simulink model "ami_fx_sbl_wide"  (R2012b)
settings: Solver=VariableStepDiscrete  SolverMode=SingleTasking  StartTime=0.0  StopTime=5000  RelTol=1e-3
undefined symbols (not defined in the file or in its folder): Down, Up
libraries: xbsIndex_r4 x4776, casper_library_misc x101, dspsigops x32, xps_library x23, casper_library_reorder x2, casper_library_delays x2
(part 8 of 43)

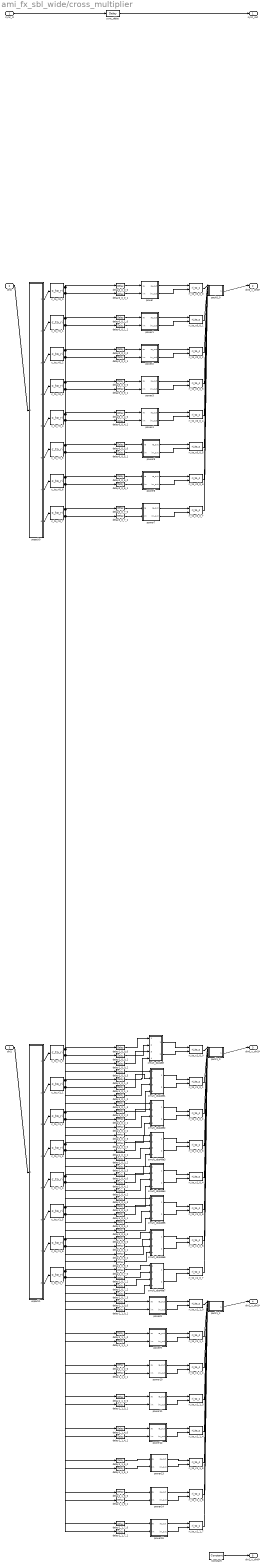
== system ami_fx_sbl_wide/cross_multiplier ==
  sync_in : Inport
  din0 : Inport  Port=2
  din1 : Inport  Port=3
  Constant : xbsIndex_r4/Constant  const=0  gui_display_data_type=Fixed-point  arith_type=Unsigned  n_bits=2*(2*bit_width_in+1)*8  bin_pt=0  preci_type=Single  exp_width=8  frac_width=24  explicit_period=on  period=1  equ=P=C  opselect=C  inp2=PCIN>>17  opr=+  inp1=P  carry=CIN  dbl_ovrd=off  block_type=constant
  c_to_ri0_{0..7} (8 alike) : casper_library_misc/c_to_ri  n_bits=bit_width_in  bin_pt=binary_point_in
  c_to_ri1_{0..7} (8 alike) : casper_library_misc/c_to_ri  n_bits=bit_width_in  bin_pt=binary_point_in
  cmult_dsp48e : Subsystem  AncestorBlock=casper_library_multipliers/cmult_dsp48e  mask(cmult_dsp48e){n_bits_a=bit_width_in, bin_pt_a=binary_point_in, n_bits_b=bit_width_in, bin_pt_b=binary_point_in, conjugated=on, full_precision=on, n_bits_c=37, bin_pt_c=34, quantization=Truncate, overflow=Wrap, cast_latency=0}
      mask prompts: n_bits_a "Bit width 'a'"; bin_pt_a "Binary point 'a'"; n_bits_b "Bit width 'b'"; bin_pt_b "Binary point 'b'"; conjugated "Conjugate"; full_precision "Full precision"; n_bits_c "Bit width out"; bin_pt_c "Binary point out"; cast_latency "Cast Latency"
      mask help:
      | Multiplies two complex numbers using 4 DSP48Es.
      | Conjugation is optional.
      |
      | Re{a} and Im{a} can be up to 25 bits.
      | Re{b} and Im{b} can be up to 18 bits.
      mask init:
      | cmult_dsp48e_init(gcb, ...
      |     'n_bits_a', n_bits_a, ...
      |     'bin_pt_a', bin_pt_a, ...
      |     'n_bits_b', n_bits_b, ...
      |     'bin_pt_b', bin_pt_b, ...
      |     'conjugated', conjugated, ...
      |     'full_precision', full_precision, ...
      |     'n_bits_c', n_bits_c, ...
      |     'bin_pt_c', bin_pt_c, ...
      |     'quantization', quantization, ...
      |     'overflow', overflow, ...
      |     'cast_latency', cast_latency);
      settings: AttributesFormatString=|
      | 18_17 * 18_17 ==> 37_34
      | Latency=4
      mask Callback full_precision:
      | full_precision = get_param(gcb, 'full_precision');
      | 
      | if strcmp(full_precision, 'on'),
      |     not_full_precision = 'off';
      | else
      |     not_full_precision = 'on';
      | end
      | 
      | set_param_state(gcb, 'n_bits_c', not_full_precision);
      | set_param_state(gcb, 'bin_pt_c', not_full_precision);
      | set_param_state(gcb, 'quantization', not_full_precision);
      | set_param_state(gcb, 'overflow', not_full_precision);
      | set_param_state(gcb, 'cast_latency', not_full_precision);
      mask TypeOptions quantization: Truncate | Round  (unbiased: +/- Inf) | Round  (unbiased: Even Values)
      mask TypeOptions overflow: Wrap | Saturate | Flag as error
  cmult_dsp48e1 : Subsystem  AncestorBlock=casper_library_multipliers/cmult_dsp48e  mask(cmult_dsp48e){n_bits_a=bit_width_in, bin_pt_a=binary_point_in, n_bits_b=bit_width_in, bin_pt_b=binary_point_in, conjugated=on, full_precision=on, n_bits_c=37, bin_pt_c=34, quantization=Truncate, overflow=Wrap, cast_latency=0}
      mask prompts: n_bits_a "Bit width 'a'"; bin_pt_a "Binary point 'a'"; n_bits_b "Bit width 'b'"; bin_pt_b "Binary point 'b'"; conjugated "Conjugate"; full_precision "Full precision"; n_bits_c "Bit width out"; bin_pt_c "Binary point out"; cast_latency "Cast Latency"
      mask help:
      | Multiplies two complex numbers using 4 DSP48Es.
      | Conjugation is optional.
      |
      | Re{a} and Im{a} can be up to 25 bits.
      | Re{b} and Im{b} can be up to 18 bits.
      mask init: same as ami_fx_sbl_wide/cross_multiplier/cmult_dsp48e
      settings: AttributesFormatString=|
      | 18_17 * 18_17 ==> 37_34
      | Latency=4
      mask Callback full_precision:
      | full_precision = get_param(gcb, 'full_precision');
      | 
      | if strcmp(full_precision, 'on'),
      |     not_full_precision = 'off';
      | else
      |     not_full_precision = 'on';
      | end
      | 
      | set_param_state(gcb, 'n_bits_c', not_full_precision);
      | set_param_state(gcb, 'bin_pt_c', not_full_precision);
      | set_param_state(gcb, 'quantization', not_full_precision);
      | set_param_state(gcb, 'overflow', not_full_precision);
      | set_param_state(gcb, 'cast_latency', not_full_precision);
      mask TypeOptions quantization: Truncate | Round  (unbiased: +/- Inf) | Round  (unbiased: Even Values)
      mask TypeOptions overflow: Wrap | Saturate | Flag as error
  cmult_dsp48e2 : Subsystem  AncestorBlock=casper_library_multipliers/cmult_dsp48e  mask(cmult_dsp48e){n_bits_a=bit_width_in, bin_pt_a=binary_point_in, n_bits_b=bit_width_in, bin_pt_b=binary_point_in, conjugated=on, full_precision=on, n_bits_c=37, bin_pt_c=34, quantization=Truncate, overflow=Wrap, cast_latency=0}
      mask prompts: n_bits_a "Bit width 'a'"; bin_pt_a "Binary point 'a'"; n_bits_b "Bit width 'b'"; bin_pt_b "Binary point 'b'"; conjugated "Conjugate"; full_precision "Full precision"; n_bits_c "Bit width out"; bin_pt_c "Binary point out"; cast_latency "Cast Latency"
      mask help:
      | Multiplies two complex numbers using 4 DSP48Es.
      | Conjugation is optional.
      |
      | Re{a} and Im{a} can be up to 25 bits.
      | Re{b} and Im{b} can be up to 18 bits.
      mask init: same as ami_fx_sbl_wide/cross_multiplier/cmult_dsp48e
      settings: AttributesFormatString=|
      | 18_17 * 18_17 ==> 37_34
      | Latency=4
      mask Callback full_precision:
      | full_precision = get_param(gcb, 'full_precision');
      | 
      | if strcmp(full_precision, 'on'),
      |     not_full_precision = 'off';
      | else
      |     not_full_precision = 'on';
      | end
      | 
      | set_param_state(gcb, 'n_bits_c', not_full_precision);
      | set_param_state(gcb, 'bin_pt_c', not_full_precision);
      | set_param_state(gcb, 'quantization', not_full_precision);
      | set_param_state(gcb, 'overflow', not_full_precision);
      | set_param_state(gcb, 'cast_latency', not_full_precision);
      mask TypeOptions quantization: Truncate | Round  (unbiased: +/- Inf) | Round  (unbiased: Even Values)
      mask TypeOptions overflow: Wrap | Saturate | Flag as error
  cmult_dsp48e3 : Subsystem  AncestorBlock=casper_library_multipliers/cmult_dsp48e  mask(cmult_dsp48e){n_bits_a=bit_width_in, bin_pt_a=binary_point_in, n_bits_b=bit_width_in, bin_pt_b=binary_point_in, conjugated=on, full_precision=on, n_bits_c=37, bin_pt_c=34, quantization=Truncate, overflow=Wrap, cast_latency=0}
      mask prompts: n_bits_a "Bit width 'a'"; bin_pt_a "Binary point 'a'"; n_bits_b "Bit width 'b'"; bin_pt_b "Binary point 'b'"; conjugated "Conjugate"; full_precision "Full precision"; n_bits_c "Bit width out"; bin_pt_c "Binary point out"; cast_latency "Cast Latency"
      mask help:
      | Multiplies two complex numbers using 4 DSP48Es.
      | Conjugation is optional.
      |
      | Re{a} and Im{a} can be up to 25 bits.
      | Re{b} and Im{b} can be up to 18 bits.
      mask init: same as ami_fx_sbl_wide/cross_multiplier/cmult_dsp48e
      settings: AttributesFormatString=|
      | 18_17 * 18_17 ==> 37_34
      | Latency=4
      mask Callback full_precision:
      | full_precision = get_param(gcb, 'full_precision');
      | 
      | if strcmp(full_precision, 'on'),
      |     not_full_precision = 'off';
      | else
      |     not_full_precision = 'on';
      | end
      | 
      | set_param_state(gcb, 'n_bits_c', not_full_precision);
      | set_param_state(gcb, 'bin_pt_c', not_full_precision);
      | set_param_state(gcb, 'quantization', not_full_precision);
      | set_param_state(gcb, 'overflow', not_full_precision);
      | set_param_state(gcb, 'cast_latency', not_full_precision);
      mask TypeOptions quantization: Truncate | Round  (unbiased: +/- Inf) | Round  (unbiased: Even Values)
      mask TypeOptions overflow: Wrap | Saturate | Flag as error
  cmult_dsp48e4 : Subsystem  AncestorBlock=casper_library_multipliers/cmult_dsp48e  mask(cmult_dsp48e){n_bits_a=bit_width_in, bin_pt_a=binary_point_in, n_bits_b=bit_width_in, bin_pt_b=binary_point_in, conjugated=on, full_precision=on, n_bits_c=37, bin_pt_c=34, quantization=Truncate, overflow=Wrap, cast_latency=0}
      mask prompts: n_bits_a "Bit width 'a'"; bin_pt_a "Binary point 'a'"; n_bits_b "Bit width 'b'"; bin_pt_b "Binary point 'b'"; conjugated "Conjugate"; full_precision "Full precision"; n_bits_c "Bit width out"; bin_pt_c "Binary point out"; cast_latency "Cast Latency"
      mask help:
      | Multiplies two complex numbers using 4 DSP48Es.
      | Conjugation is optional.
      |
      | Re{a} and Im{a} can be up to 25 bits.
      | Re{b} and Im{b} can be up to 18 bits.
      mask init: same as ami_fx_sbl_wide/cross_multiplier/cmult_dsp48e
      settings: AttributesFormatString=|
      | 18_17 * 18_17 ==> 37_34
      | Latency=4
      mask Callback full_precision:
      | full_precision = get_param(gcb, 'full_precision');
      | 
      | if strcmp(full_precision, 'on'),
      |     not_full_precision = 'off';
      | else
      |     not_full_precision = 'on';
      | end
      | 
      | set_param_state(gcb, 'n_bits_c', not_full_precision);
      | set_param_state(gcb, 'bin_pt_c', not_full_precision);
      | set_param_state(gcb, 'quantization', not_full_precision);
      | set_param_state(gcb, 'overflow', not_full_precision);
      | set_param_state(gcb, 'cast_latency', not_full_precision);
      mask TypeOptions quantization: Truncate | Round  (unbiased: +/- Inf) | Round  (unbiased: Even Values)
      mask TypeOptions overflow: Wrap | Saturate | Flag as error
  cmult_dsp48e5 : Subsystem  AncestorBlock=casper_library_multipliers/cmult_dsp48e  mask(cmult_dsp48e){n_bits_a=bit_width_in, bin_pt_a=binary_point_in, n_bits_b=bit_width_in, bin_pt_b=binary_point_in, conjugated=on, full_precision=on, n_bits_c=37, bin_pt_c=34, quantization=Truncate, overflow=Wrap, cast_latency=0}
      mask prompts: n_bits_a "Bit width 'a'"; bin_pt_a "Binary point 'a'"; n_bits_b "Bit width 'b'"; bin_pt_b "Binary point 'b'"; conjugated "Conjugate"; full_precision "Full precision"; n_bits_c "Bit width out"; bin_pt_c "Binary point out"; cast_latency "Cast Latency"
      mask help:
      | Multiplies two complex numbers using 4 DSP48Es.
      | Conjugation is optional.
      |
      | Re{a} and Im{a} can be up to 25 bits.
      | Re{b} and Im{b} can be up to 18 bits.
      mask init: same as ami_fx_sbl_wide/cross_multiplier/cmult_dsp48e
      settings: AttributesFormatString=|
      | 18_17 * 18_17 ==> 37_34
      | Latency=4
      mask Callback full_precision:
      | full_precision = get_param(gcb, 'full_precision');
      | 
      | if strcmp(full_precision, 'on'),
      |     not_full_precision = 'off';
      | else
      |     not_full_precision = 'on';
      | end
      | 
      | set_param_state(gcb, 'n_bits_c', not_full_precision);
      | set_param_state(gcb, 'bin_pt_c', not_full_precision);
      | set_param_state(gcb, 'quantization', not_full_precision);
      | set_param_state(gcb, 'overflow', not_full_precision);
      | set_param_state(gcb, 'cast_latency', not_full_precision);
      mask TypeOptions quantization: Truncate | Round  (unbiased: +/- Inf) | Round  (unbiased: Even Values)
      mask TypeOptions overflow: Wrap | Saturate | Flag as error
  cmult_dsp48e6 : Subsystem  AncestorBlock=casper_library_multipliers/cmult_dsp48e  mask(cmult_dsp48e){n_bits_a=bit_width_in, bin_pt_a=binary_point_in, n_bits_b=bit_width_in, bin_pt_b=binary_point_in, conjugated=on, full_precision=on, n_bits_c=37, bin_pt_c=34, quantization=Truncate, overflow=Wrap, cast_latency=0}
      mask prompts: n_bits_a "Bit width 'a'"; bin_pt_a "Binary point 'a'"; n_bits_b "Bit width 'b'"; bin_pt_b "Binary point 'b'"; conjugated "Conjugate"; full_precision "Full precision"; n_bits_c "Bit width out"; bin_pt_c "Binary point out"; cast_latency "Cast Latency"
      mask help:
      | Multiplies two complex numbers using 4 DSP48Es.
      | Conjugation is optional.
      |
      | Re{a} and Im{a} can be up to 25 bits.
      | Re{b} and Im{b} can be up to 18 bits.
      mask init: same as ami_fx_sbl_wide/cross_multiplier/cmult_dsp48e
      settings: AttributesFormatString=|
      | 18_17 * 18_17 ==> 37_34
      | Latency=4
      mask Callback full_precision:
      | full_precision = get_param(gcb, 'full_precision');
      | 
      | if strcmp(full_precision, 'on'),
      |     not_full_precision = 'off';
      | else
      |     not_full_precision = 'on';
      | end
      | 
      | set_param_state(gcb, 'n_bits_c', not_full_precision);
      | set_param_state(gcb, 'bin_pt_c', not_full_precision);
      | set_param_state(gcb, 'quantization', not_full_precision);
      | set_param_state(gcb, 'overflow', not_full_precision);
      | set_param_state(gcb, 'cast_latency', not_full_precision);
      mask TypeOptions quantization: Truncate | Round  (unbiased: +/- Inf) | Round  (unbiased: Even Values)
      mask TypeOptions overflow: Wrap | Saturate | Flag as error
  cmult_dsp48e7 : Subsystem  AncestorBlock=casper_library_multipliers/cmult_dsp48e  mask(cmult_dsp48e){n_bits_a=bit_width_in, bin_pt_a=binary_point_in, n_bits_b=bit_width_in, bin_pt_b=binary_point_in, conjugated=on, full_precision=on, n_bits_c=37, bin_pt_c=34, quantization=Truncate, overflow=Wrap, cast_latency=0}
      mask prompts: n_bits_a "Bit width 'a'"; bin_pt_a "Binary point 'a'"; n_bits_b "Bit width 'b'"; bin_pt_b "Binary point 'b'"; conjugated "Conjugate"; full_precision "Full precision"; n_bits_c "Bit width out"; bin_pt_c "Binary point out"; cast_latency "Cast Latency"
      mask help:
      | Multiplies two complex numbers using 4 DSP48Es.
      | Conjugation is optional.
      |
      | Re{a} and Im{a} can be up to 25 bits.
      | Re{b} and Im{b} can be up to 18 bits.
      mask init: same as ami_fx_sbl_wide/cross_multiplier/cmult_dsp48e
      settings: AttributesFormatString=|
      | 18_17 * 18_17 ==> 37_34
      | Latency=4
      mask Callback full_precision:
      | full_precision = get_param(gcb, 'full_precision');
      | 
      | if strcmp(full_precision, 'on'),
      |     not_full_precision = 'off';
      | else
      |     not_full_precision = 'on';
      | end
      | 
      | set_param_state(gcb, 'n_bits_c', not_full_precision);
      | set_param_state(gcb, 'bin_pt_c', not_full_precision);
      | set_param_state(gcb, 'quantization', not_full_precision);
      | set_param_state(gcb, 'overflow', not_full_precision);
      | set_param_state(gcb, 'cast_latency', not_full_precision);
      mask TypeOptions quantization: Truncate | Round  (unbiased: +/- Inf) | Round  (unbiased: Even Values)
      mask TypeOptions overflow: Wrap | Saturate | Flag as error
  delay0_0_0_0 : xbsIndex_r4/Delay  rst=off  infoeditControl=Selection of Reset will increase slice count due to use of real FFs and instead of SRLs  en=off  latency=1  dbl_ovrd=off  reg_retiming=off  block_type=delay
  delay0_0_0_1 : xbsIndex_r4/Delay  rst=off  infoeditControl=Selection of Reset will increase slice count due to use of real FFs and instead of SRLs  en=off  latency=1  dbl_ovrd=off  reg_retiming=off  block_type=delay
  delay0_0_1_0 : xbsIndex_r4/Delay  rst=off  infoeditControl=Selection of Reset will increase slice count due to use of real FFs and instead of SRLs  en=off  latency=1  dbl_ovrd=off  reg_retiming=off  block_type=delay
  delay0_0_1_1 : xbsIndex_r4/Delay  rst=off  infoeditControl=Selection of Reset will increase slice count due to use of real FFs and instead of SRLs  en=off  latency=1  dbl_ovrd=off  reg_retiming=off  block_type=delay
  delay0_0_2_0 : xbsIndex_r4/Delay  rst=off  infoeditControl=Selection of Reset will increase slice count due to use of real FFs and instead of SRLs  en=off  latency=1  dbl_ovrd=off  reg_retiming=off  block_type=delay
  delay0_0_2_1 : xbsIndex_r4/Delay  rst=off  infoeditControl=Selection of Reset will increase slice count due to use of real FFs and instead of SRLs  en=off  latency=1  dbl_ovrd=off  reg_retiming=off  block_type=delay
  delay0_0_3_0 : xbsIndex_r4/Delay  rst=off  infoeditControl=Selection of Reset will increase slice count due to use of real FFs and instead of SRLs  en=off  latency=1  dbl_ovrd=off  reg_retiming=off  block_type=delay
  delay0_0_3_1 : xbsIndex_r4/Delay  rst=off  infoeditControl=Selection of Reset will increase slice count due to use of real FFs and instead of SRLs  en=off  latency=1  dbl_ovrd=off  reg_retiming=off  block_type=delay
  delay0_0_4_0 : xbsIndex_r4/Delay  rst=off  infoeditControl=Selection of Reset will increase slice count due to use of real FFs and instead of SRLs  en=off  latency=1  dbl_ovrd=off  reg_retiming=off  block_type=delay
  delay0_0_4_1 : xbsIndex_r4/Delay  rst=off  infoeditControl=Selection of Reset will increase slice count due to use of real FFs and instead of SRLs  en=off  latency=1  dbl_ovrd=off  reg_retiming=off  block_type=delay
  delay0_0_5_0 : xbsIndex_r4/Delay  rst=off  infoeditControl=Selection of Reset will increase slice count due to use of real FFs and instead of SRLs  en=off  latency=1  dbl_ovrd=off  reg_retiming=off  block_type=delay
  delay0_0_5_1 : xbsIndex_r4/Delay  rst=off  infoeditControl=Selection of Reset will increase slice count due to use of real FFs and instead of SRLs  en=off  latency=1  dbl_ovrd=off  reg_retiming=off  block_type=delay
  delay0_0_6_0 : xbsIndex_r4/Delay  rst=off  infoeditControl=Selection of Reset will increase slice count due to use of real FFs and instead of SRLs  en=off  latency=1  dbl_ovrd=off  reg_retiming=off  block_type=delay
  delay0_0_6_1 : xbsIndex_r4/Delay  rst=off  infoeditControl=Selection of Reset will increase slice count due to use of real FFs and instead of SRLs  en=off  latency=1  dbl_ovrd=off  reg_retiming=off  block_type=delay
  delay0_0_7_0 : xbsIndex_r4/Delay  rst=off  infoeditControl=Selection of Reset will increase slice count due to use of real FFs and instead of SRLs  en=off  latency=1  dbl_ovrd=off  reg_retiming=off  block_type=delay
  delay0_0_7_1 : xbsIndex_r4/Delay  rst=off  infoeditControl=Selection of Reset will increase slice count due to use of real FFs and instead of SRLs  en=off  latency=1  dbl_ovrd=off  reg_retiming=off  block_type=delay
  delay1_0_0_{0..3} (4 alike) : xbsIndex_r4/Delay  rst=off  infoeditControl=Selection of Reset will increase slice count due to use of real FFs and instead of SRLs  en=off  latency=1  dbl_ovrd=off  reg_retiming=off  block_type=delay
  delay1_0_1_{0..3} (4 alike) : xbsIndex_r4/Delay  rst=off  infoeditControl=Selection of Reset will increase slice count due to use of real FFs and instead of SRLs  en=off  latency=1  dbl_ovrd=off  reg_retiming=off  block_type=delay
  delay1_0_2_{0..3} (4 alike) : xbsIndex_r4/Delay  rst=off  infoeditControl=Selection of Reset will increase slice count due to use of real FFs and instead of SRLs  en=off  latency=1  dbl_ovrd=off  reg_retiming=off  block_type=delay
  delay1_0_3_{0..3} (4 alike) : xbsIndex_r4/Delay  rst=off  infoeditControl=Selection of Reset will increase slice count due to use of real FFs and instead of SRLs  en=off  latency=1  dbl_ovrd=off  reg_retiming=off  block_type=delay
  delay1_0_4_{0..3} (4 alike) : xbsIndex_r4/Delay  rst=off  infoeditControl=Selection of Reset will increase slice count due to use of real FFs and instead of SRLs  en=off  latency=1  dbl_ovrd=off  reg_retiming=off  block_type=delay
  delay1_0_5_{0..3} (4 alike) : xbsIndex_r4/Delay  rst=off  infoeditControl=Selection of Reset will increase slice count due to use of real FFs and instead of SRLs  en=off  latency=1  dbl_ovrd=off  reg_retiming=off  block_type=delay
  delay1_0_6_{0..3} (4 alike) : xbsIndex_r4/Delay  rst=off  infoeditControl=Selection of Reset will increase slice count due to use of real FFs and instead of SRLs  en=off  latency=1  dbl_ovrd=off  reg_retiming=off  block_type=delay
  delay1_0_7_{0..3} (4 alike) : xbsIndex_r4/Delay  rst=off  infoeditControl=Selection of Reset will increase slice count due to use of real FFs and instead of SRLs  en=off  latency=1  dbl_ovrd=off  reg_retiming=off  block_type=delay
  delay1_1_0_0 : xbsIndex_r4/Delay  rst=off  infoeditControl=Selection of Reset will increase slice count due to use of real FFs and instead of SRLs  en=off  latency=1  dbl_ovrd=off  reg_retiming=off  block_type=delay
  delay1_1_0_1 : xbsIndex_r4/Delay  rst=off  infoeditControl=Selection of Reset will increase slice count due to use of real FFs and instead of SRLs  en=off  latency=1  dbl_ovrd=off  reg_retiming=off  block_type=delay
  delay1_1_1_0 : xbsIndex_r4/Delay  rst=off  infoeditControl=Selection of Reset will increase slice count due to use of real FFs and instead of SRLs  en=off  latency=1  dbl_ovrd=off  reg_retiming=off  block_type=delay
  delay1_1_1_1 : xbsIndex_r4/Delay  rst=off  infoeditControl=Selection of Reset will increase slice count due to use of real FFs and instead of SRLs  en=off  latency=1  dbl_ovrd=off  reg_retiming=off  block_type=delay
  delay1_1_2_0 : xbsIndex_r4/Delay  rst=off  infoeditControl=Selection of Reset will increase slice count due to use of real FFs and instead of SRLs  en=off  latency=1  dbl_ovrd=off  reg_retiming=off  block_type=delay
  delay1_1_2_1 : xbsIndex_r4/Delay  rst=off  infoeditControl=Selection of Reset will increase slice count due to use of real FFs and instead of SRLs  en=off  latency=1  dbl_ovrd=off  reg_retiming=off  block_type=delay
  delay1_1_3_0 : xbsIndex_r4/Delay  rst=off  infoeditControl=Selection of Reset will increase slice count due to use of real FFs and instead of SRLs  en=off  latency=1  dbl_ovrd=off  reg_retiming=off  block_type=delay
  delay1_1_3_1 : xbsIndex_r4/Delay  rst=off  infoeditControl=Selection of Reset will increase slice count due to use of real FFs and instead of SRLs  en=off  latency=1  dbl_ovrd=off  reg_retiming=off  block_type=delay
  delay1_1_4_0 : xbsIndex_r4/Delay  rst=off  infoeditControl=Selection of Reset will increase slice count due to use of real FFs and instead of SRLs  en=off  latency=1  dbl_ovrd=off  reg_retiming=off  block_type=delay
  delay1_1_4_1 : xbsIndex_r4/Delay  rst=off  infoeditControl=Selection of Reset will increase slice count due to use of real FFs and instead of SRLs  en=off  latency=1  dbl_ovrd=off  reg_retiming=off  block_type=delay
  delay1_1_5_0 : xbsIndex_r4/Delay  rst=off  infoeditControl=Selection of Reset will increase slice count due to use of real FFs and instead of SRLs  en=off  latency=1  dbl_ovrd=off  reg_retiming=off  block_type=delay
  delay1_1_5_1 : xbsIndex_r4/Delay  rst=off  infoeditControl=Selection of Reset will increase slice count due to use of real FFs and instead of SRLs  en=off  latency=1  dbl_ovrd=off  reg_retiming=off  block_type=delay
  delay1_1_6_0 : xbsIndex_r4/Delay  rst=off  infoeditControl=Selection of Reset will increase slice count due to use of real FFs and instead of SRLs  en=off  latency=1  dbl_ovrd=off  reg_retiming=off  block_type=delay
  delay1_1_6_1 : xbsIndex_r4/Delay  rst=off  infoeditControl=Selection of Reset will increase slice count due to use of real FFs and instead of SRLs  en=off  latency=1  dbl_ovrd=off  reg_retiming=off  block_type=delay
  delay1_1_7_0 : xbsIndex_r4/Delay  rst=off  infoeditControl=Selection of Reset will increase slice count due to use of real FFs and instead of SRLs  en=off  latency=1  dbl_ovrd=off  reg_retiming=off  block_type=delay
  delay1_1_7_1 : xbsIndex_r4/Delay  rst=off  infoeditControl=Selection of Reset will increase slice count due to use of real FFs and instead of SRLs  en=off  latency=1  dbl_ovrd=off  reg_retiming=off  block_type=delay
  pack0_0 : Subsystem  AncestorBlock=casper_library_flow_control/bus_create  mask(bus_create){inputNum=aggregation}
      mask prompts: inputNum "Number of inputs:"
      mask init:
      | bus_create_init(gcb,...
      |     'inputNum', inputNum);
  pack1_0 : Subsystem  AncestorBlock=casper_library_flow_control/bus_create  mask(bus_create){inputNum=aggregation}
      mask prompts: inputNum "Number of inputs:"
      mask init:
      | bus_create_init(gcb,...
      |     'inputNum', inputNum);
  pack1_1 : Subsystem  AncestorBlock=casper_library_flow_control/bus_create  mask(bus_create){inputNum=aggregation}
      mask prompts: inputNum "Number of inputs:"
      mask init:
      | bus_create_init(gcb,...
      |     'inputNum', inputNum);
  power : Subsystem  mask{bit_width_in=bit_width_in, binary_pt_in=binary_point_in}
      mask prompts: bit_width_in "bit width in?"; binary_pt_in "binary point in?"
  power1 : Subsystem  mask{bit_width_in=bit_width_in, binary_pt_in=binary_point_in}
      mask prompts: bit_width_in "bit width in?"; binary_pt_in "binary point in?"
  power10 : Subsystem  mask{bit_width_in=bit_width_in, binary_pt_in=binary_point_in}
      mask prompts: bit_width_in "bit width in?"; binary_pt_in "binary point in?"
  power11 : Subsystem  mask{bit_width_in=bit_width_in, binary_pt_in=binary_point_in}
      mask prompts: bit_width_in "bit width in?"; binary_pt_in "binary point in?"
  power12 : Subsystem  mask{bit_width_in=bit_width_in, binary_pt_in=binary_point_in}
      mask prompts: bit_width_in "bit width in?"; binary_pt_in "binary point in?"
  power13 : Subsystem  mask{bit_width_in=bit_width_in, binary_pt_in=binary_point_in}
      mask prompts: bit_width_in "bit width in?"; binary_pt_in "binary point in?"
  power14 : Subsystem  mask{bit_width_in=bit_width_in, binary_pt_in=binary_point_in}
      mask prompts: bit_width_in "bit width in?"; binary_pt_in "binary point in?"
  power15 : Subsystem  mask{bit_width_in=bit_width_in, binary_pt_in=binary_point_in}
      mask prompts: bit_width_in "bit width in?"; binary_pt_in "binary point in?"
  power2 : Subsystem  mask{bit_width_in=bit_width_in, binary_pt_in=binary_point_in}
      mask prompts: bit_width_in "bit width in?"; binary_pt_in "binary point in?"
  power3 : Subsystem  mask{bit_width_in=bit_width_in, binary_pt_in=binary_point_in}
      mask prompts: bit_width_in "bit width in?"; binary_pt_in "binary point in?"
  power4 : Subsystem  mask{bit_width_in=bit_width_in, binary_pt_in=binary_point_in}
      mask prompts: bit_width_in "bit width in?"; binary_pt_in "binary point in?"
  power5 : Subsystem  mask{bit_width_in=bit_width_in, binary_pt_in=binary_point_in}
      mask prompts: bit_width_in "bit width in?"; binary_pt_in "binary point in?"
  power6 : Subsystem  mask{bit_width_in=bit_width_in, binary_pt_in=binary_point_in}
      mask prompts: bit_width_in "bit width in?"; binary_pt_in "binary point in?"
  power7 : Subsystem  mask{bit_width_in=bit_width_in, binary_pt_in=binary_point_in}
      mask prompts: bit_width_in "bit width in?"; binary_pt_in "binary point in?"
  power8 : Subsystem  mask{bit_width_in=bit_width_in, binary_pt_in=binary_point_in}
      mask prompts: bit_width_in "bit width in?"; binary_pt_in "binary point in?"
  power9 : Subsystem  mask{bit_width_in=bit_width_in, binary_pt_in=binary_point_in}
      mask prompts: bit_width_in "bit width in?"; binary_pt_in "binary point in?"
  ri_to_c0_0_{0..7} (8 alike) : casper_library_misc/ri_to_c
  ri_to_c1_0_{0..7} (8 alike) : casper_library_misc/ri_to_c
  ri_to_c1_1_{0..7} (8 alike) : casper_library_misc/ri_to_c
  sync_delay : xbsIndex_r4/Delay  rst=off  infoeditControl=Selection of Reset will increase slice count due to use of real FFs and instead of SRLs  en=off  latency=mult_latency+add_latency+1+conv_latency  dbl_ovrd=off  reg_retiming=off  block_type=delay
  unpack0 : Subsystem  AncestorBlock=casper_library_flow_control/bus_expand  mask(bus_expand){mode=divisions of equal size, outputNum=aggregation, outputWidth=bit_width_in*2, outputBinaryPt=0, outputArithmeticType=0, show_format=off, outputToWorkspace=off, variablePrefix=out, outputToModelAsWell=on}
      mask prompts: outputNum "Number of outputs:"; outputWidth "Output width:"; outputBinaryPt "Output binary point position:"; outputArithmeticType "Output arithmetic type (ufix=0, fix=1, bool=2):"; show_format "Print format string?"; outputToWorkspace "Output to workspace?"; variablePrefix "Variable name prefix:"; outputToModelAsWell "Output to model as well?"
      mask help:
      | Expands a 'bus' made using a bus_create or Xilinx
      | concat block.
      | The input will be divided into the specified number
      | of outputs with the specified arithmetic types.
      | Divisions are made from most significant bit.
      mask init: same as ami_fx_sbl_wide/bus_expand
      settings: AttributesFormatString=8 outputs
      mask TypeOptions mode: divisions of equal size | divisions of arbitrary size
      mask Callback mode: bus_expand_callback();
      mask Callback outputWidth: bus_expand_callback();
      mask Callback outputToWorkspace: bus_expand_callback();
  unpack1 : Subsystem  AncestorBlock=casper_library_flow_control/bus_expand  mask(bus_expand){mode=divisions of equal size, outputNum=aggregation, outputWidth=bit_width_in*2, outputBinaryPt=0, outputArithmeticType=0, show_format=off, outputToWorkspace=off, variablePrefix=out, outputToModelAsWell=on}
      mask prompts: outputNum "Number of outputs:"; outputWidth "Output width:"; outputBinaryPt "Output binary point position:"; outputArithmeticType "Output arithmetic type (ufix=0, fix=1, bool=2):"; show_format "Print format string?"; outputToWorkspace "Output to workspace?"; variablePrefix "Variable name prefix:"; outputToModelAsWell "Output to model as well?"
      mask help:
      | Expands a 'bus' made using a bus_create or Xilinx
      | concat block.
      | The input will be divided into the specified number
      | of outputs with the specified arithmetic types.
      | Divisions are made from most significant bit.
      mask init: same as ami_fx_sbl_wide/bus_expand
      settings: AttributesFormatString=8 outputs
      mask TypeOptions mode: divisions of equal size | divisions of arbitrary size
      mask Callback mode: bus_expand_callback();
      mask Callback outputWidth: bus_expand_callback();
      mask Callback outputToWorkspace: bus_expand_callback();
  sync_out : Outport
  din0_x_din0* : Outport  Port=2
  din0_x_din1* : Outport  Port=3
  din1_x_din1* : Outport  Port=4
  din1_x_din0* : Outport  Port=5
  wires:
  sync_in/1 -> sync_delay/1
  sync_delay/1 -> sync_out/1
  din0/1 -> unpack0/1(bus_in)
  unpack0/1(msb_out8) -> c_to_ri0_0/1
  unpack0/2(out7) -> c_to_ri0_1/1
  unpack0/3(out6) -> c_to_ri0_2/1
  unpack0/4(out5) -> c_to_ri0_3/1
  unpack0/5(out4) -> c_to_ri0_4/1
  unpack0/6(out3) -> c_to_ri0_5/1
  unpack0/7(out2) -> c_to_ri0_6/1
  unpack0/8(lsb_out1) -> c_to_ri0_7/1
  c_to_ri0_0/1 -> delay0_0_0_0/1, delay1_0_0_0/1
  c_to_ri0_0/2 -> delay0_0_0_1/1, delay1_0_0_1/1
  ri_to_c0_0_0/1 -> pack0_0/1(in1)
  c_to_ri0_1/1 -> delay0_0_1_0/1, delay1_0_1_0/1
  c_to_ri0_1/2 -> delay0_0_1_1/1, delay1_0_1_1/1
  ri_to_c0_0_1/1 -> pack0_0/2(in2)
  c_to_ri0_2/1 -> delay0_0_2_0/1, delay1_0_2_0/1
  c_to_ri0_2/2 -> delay0_0_2_1/1, delay1_0_2_1/1
  ri_to_c0_0_2/1 -> pack0_0/3(in3)
  c_to_ri0_3/1 -> delay0_0_3_0/1, delay1_0_3_0/1
  c_to_ri0_3/2 -> delay0_0_3_1/1, delay1_0_3_1/1
  ri_to_c0_0_3/1 -> pack0_0/4(in4)
  c_to_ri0_4/1 -> delay0_0_4_0/1, delay1_0_4_0/1
  c_to_ri0_4/2 -> delay0_0_4_1/1, delay1_0_4_1/1
  ri_to_c0_0_4/1 -> pack0_0/5(in5)
  c_to_ri0_5/1 -> delay0_0_5_0/1, delay1_0_5_0/1
  c_to_ri0_5/2 -> delay0_0_5_1/1, delay1_0_5_1/1
  ri_to_c0_0_5/1 -> pack0_0/6(in6)
  c_to_ri0_6/1 -> delay0_0_6_0/1, delay1_0_6_0/1
  c_to_ri0_6/2 -> delay0_0_6_1/1, delay1_0_6_1/1
  ri_to_c0_0_6/1 -> pack0_0/7(in7)
  c_to_ri0_7/1 -> delay0_0_7_0/1, delay1_0_7_0/1
  c_to_ri0_7/2 -> delay0_0_7_1/1, delay1_0_7_1/1
  ri_to_c0_0_7/1 -> pack0_0/8(in8)
  pack0_0/1(bus_out) -> din0_x_din0*/1
  din1/1 -> unpack1/1(bus_in)
  unpack1/1(msb_out8) -> c_to_ri1_0/1
  unpack1/2(out7) -> c_to_ri1_1/1
  unpack1/3(out6) -> c_to_ri1_2/1
  unpack1/4(out5) -> c_to_ri1_3/1
  unpack1/5(out4) -> c_to_ri1_4/1
  unpack1/6(out3) -> c_to_ri1_5/1
  unpack1/7(out2) -> c_to_ri1_6/1
  unpack1/8(lsb_out1) -> c_to_ri1_7/1
  c_to_ri1_0/1 -> delay1_0_0_2/1, delay1_1_0_0/1
  c_to_ri1_0/2 -> delay1_0_0_3/1, delay1_1_0_1/1
  ri_to_c1_0_0/1 -> pack1_0/1(in1)
  c_to_ri1_1/1 -> delay1_0_1_2/1, delay1_1_1_0/1
  c_to_ri1_1/2 -> delay1_0_1_3/1, delay1_1_1_1/1
  ri_to_c1_0_1/1 -> pack1_0/2(in2)
  c_to_ri1_2/1 -> delay1_0_2_2/1, delay1_1_2_0/1
  c_to_ri1_2/2 -> delay1_0_2_3/1, delay1_1_2_1/1
  ri_to_c1_0_2/1 -> pack1_0/3(in3)
  c_to_ri1_3/1 -> delay1_0_3_2/1, delay1_1_3_0/1
  c_to_ri1_3/2 -> delay1_0_3_3/1, delay1_1_3_1/1
  ri_to_c1_0_3/1 -> pack1_0/4(in4)
  c_to_ri1_4/1 -> delay1_0_4_2/1, delay1_1_4_0/1
  c_to_ri1_4/2 -> delay1_0_4_3/1, delay1_1_4_1/1
  ri_to_c1_0_4/1 -> pack1_0/5(in5)
  c_to_ri1_5/1 -> delay1_0_5_2/1, delay1_1_5_0/1
  c_to_ri1_5/2 -> delay1_0_5_3/1, delay1_1_5_1/1
  ri_to_c1_0_5/1 -> pack1_0/6(in6)
  c_to_ri1_6/1 -> delay1_0_6_2/1, delay1_1_6_0/1
  c_to_ri1_6/2 -> delay1_0_6_3/1, delay1_1_6_1/1
  ri_to_c1_0_6/1 -> pack1_0/7(in7)
  c_to_ri1_7/1 -> delay1_0_7_2/1, delay1_1_7_0/1
  c_to_ri1_7/2 -> delay1_0_7_3/1, delay1_1_7_1/1
  ri_to_c1_0_7/1 -> pack1_0/8(in8)
  pack1_0/1(bus_out) -> din0_x_din1*/1
  ri_to_c1_1_0/1 -> pack1_1/1(in1)
  ri_to_c1_1_1/1 -> pack1_1/2(in2)
  ri_to_c1_1_2/1 -> pack1_1/3(in3)
  ri_to_c1_1_3/1 -> pack1_1/4(in4)
  ri_to_c1_1_4/1 -> pack1_1/5(in5)
  ri_to_c1_1_5/1 -> pack1_1/6(in6)
  ri_to_c1_1_6/1 -> pack1_1/7(in7)
  ri_to_c1_1_7/1 -> pack1_1/8(in8)
  pack1_1/1(bus_out) -> din1_x_din1*/1
  delay0_0_0_0/1 -> power/1(re)
  delay0_0_0_1/1 -> power/2(im)
  power/1(re_out) -> ri_to_c0_0_0/1
  power/2(im_out) -> ri_to_c0_0_0/2
  delay0_0_1_1/1 -> power1/2(im)
  delay0_0_1_0/1 -> power1/1(re)
  power1/1(re_out) -> ri_to_c0_0_1/1
  power1/2(im_out) -> ri_to_c0_0_1/2
  delay0_0_2_0/1 -> power2/1(re)
  delay0_0_2_1/1 -> power2/2(im)
  power2/1(re_out) -> ri_to_c0_0_2/1
  power2/2(im_out) -> ri_to_c0_0_2/2
  delay0_0_3_0/1 -> power3/1(re)
  delay0_0_3_1/1 -> power3/2(im)
  power3/1(re_out) -> ri_to_c0_0_3/1
  power3/2(im_out) -> ri_to_c0_0_3/2
  delay0_0_4_0/1 -> power4/1(re)
  delay0_0_4_1/1 -> power4/2(im)
  power4/1(re_out) -> ri_to_c0_0_4/1
  power4/2(im_out) -> ri_to_c0_0_4/2
  delay0_0_5_0/1 -> power5/1(re)
  delay0_0_5_1/1 -> power5/2(im)
  power5/1(re_out) -> ri_to_c0_0_5/1
  power5/2(im_out) -> ri_to_c0_0_5/2
  delay0_0_6_0/1 -> power6/1(re)
  delay0_0_6_1/1 -> power6/2(im)
  power6/1(re_out) -> ri_to_c0_0_6/1
  power6/2(im_out) -> ri_to_c0_0_6/2
  power7/1(re_out) -> ri_to_c0_0_7/1
  power7/2(im_out) -> ri_to_c0_0_7/2
  delay0_0_7_1/1 -> power7/2(im)
  delay0_0_7_0/1 -> power7/1(re)
  delay1_0_0_0/1 -> cmult_dsp48e/1(a_re)
  delay1_0_0_1/1 -> cmult_dsp48e/2(a_im)
  delay1_0_0_2/1 -> cmult_dsp48e/3(b_re)
  delay1_0_0_3/1 -> cmult_dsp48e/4(b_im)
  cmult_dsp48e/2(c_im) -> ri_to_c1_0_0/2
  cmult_dsp48e/1(c_re) -> ri_to_c1_0_0/1
  delay1_0_1_0/1 -> cmult_dsp48e1/1(a_re)
  delay1_0_1_1/1 -> cmult_dsp48e1/2(a_im)
  delay1_0_1_2/1 -> cmult_dsp48e1/3(b_re)
  delay1_0_1_3/1 -> cmult_dsp48e1/4(b_im)
  cmult_dsp48e1/1(c_re) -> ri_to_c1_0_1/1
  cmult_dsp48e1/2(c_im) -> ri_to_c1_0_1/2
  delay1_0_2_0/1 -> cmult_dsp48e2/1(a_re)
  delay1_0_2_1/1 -> cmult_dsp48e2/2(a_im)
  delay1_0_2_2/1 -> cmult_dsp48e2/3(b_re)
  delay1_0_2_3/1 -> cmult_dsp48e2/4(b_im)
  cmult_dsp48e2/1(c_re) -> ri_to_c1_0_2/1
  cmult_dsp48e2/2(c_im) -> ri_to_c1_0_2/2
  delay1_0_3_0/1 -> cmult_dsp48e3/1(a_re)
  delay1_0_3_1/1 -> cmult_dsp48e3/2(a_im)
  delay1_0_3_2/1 -> cmult_dsp48e3/3(b_re)
  delay1_0_3_3/1 -> cmult_dsp48e3/4(b_im)
  cmult_dsp48e3/1(c_re) -> ri_to_c1_0_3/1
  cmult_dsp48e3/2(c_im) -> ri_to_c1_0_3/2
  delay1_0_4_0/1 -> cmult_dsp48e4/1(a_re)
  delay1_0_4_1/1 -> cmult_dsp48e4/2(a_im)
  delay1_0_4_2/1 -> cmult_dsp48e4/3(b_re)
  delay1_0_4_3/1 -> cmult_dsp48e4/4(b_im)
  cmult_dsp48e4/1(c_re) -> ri_to_c1_0_4/1
  cmult_dsp48e4/2(c_im) -> ri_to_c1_0_4/2
  delay1_0_5_0/1 -> cmult_dsp48e5/1(a_re)
  delay1_0_5_1/1 -> cmult_dsp48e5/2(a_im)
  delay1_0_5_2/1 -> cmult_dsp48e5/3(b_re)
  delay1_0_5_3/1 -> cmult_dsp48e5/4(b_im)
  cmult_dsp48e5/1(c_re) -> ri_to_c1_0_5/1
  cmult_dsp48e5/2(c_im) -> ri_to_c1_0_5/2
  delay1_0_6_0/1 -> cmult_dsp48e6/1(a_re)
  delay1_0_6_1/1 -> cmult_dsp48e6/2(a_im)
  delay1_0_6_2/1 -> cmult_dsp48e6/3(b_re)
  delay1_0_6_3/1 -> cmult_dsp48e6/4(b_im)
  cmult_dsp48e6/1(c_re) -> ri_to_c1_0_6/1
  cmult_dsp48e6/2(c_im) -> ri_to_c1_0_6/2
  delay1_0_7_0/1 -> cmult_dsp48e7/1(a_re)
  delay1_0_7_1/1 -> cmult_dsp48e7/2(a_im)
  delay1_0_7_2/1 -> cmult_dsp48e7/3(b_re)
  delay1_0_7_3/1 -> cmult_dsp48e7/4(b_im)
  cmult_dsp48e7/1(c_re) -> ri_to_c1_0_7/1
  cmult_dsp48e7/2(c_im) -> ri_to_c1_0_7/2
  delay1_1_0_0/1 -> power8/1(re)
  delay1_1_0_1/1 -> power8/2(im)
  power8/1(re_out) -> ri_to_c1_1_0/1
  power8/2(im_out) -> ri_to_c1_1_0/2
  delay1_1_1_0/1 -> power9/1(re)
  delay1_1_1_1/1 -> power9/2(im)
  power9/1(re_out) -> ri_to_c1_1_1/1
  power9/2(im_out) -> ri_to_c1_1_1/2
  delay1_1_2_0/1 -> power10/1(re)
  delay1_1_2_1/1 -> power10/2(im)
  power10/1(re_out) -> ri_to_c1_1_2/1
  power10/2(im_out) -> ri_to_c1_1_2/2
  delay1_1_3_0/1 -> power11/1(re)
  delay1_1_3_1/1 -> power11/2(im)
  power11/1(re_out) -> ri_to_c1_1_3/1
  power11/2(im_out) -> ri_to_c1_1_3/2
  delay1_1_4_0/1 -> power12/1(re)
  delay1_1_4_1/1 -> power12/2(im)
  power12/1(re_out) -> ri_to_c1_1_4/1
  power12/2(im_out) -> ri_to_c1_1_4/2
  delay1_1_5_0/1 -> power13/1(re)
  delay1_1_5_1/1 -> power13/2(im)
  power13/1(re_out) -> ri_to_c1_1_5/1
  power13/2(im_out) -> ri_to_c1_1_5/2
  delay1_1_6_1/1 -> power14/2(im)
  delay1_1_6_0/1 -> power14/1(re)
  power14/1(re_out) -> ri_to_c1_1_6/1
  power14/2(im_out) -> ri_to_c1_1_6/2
  delay1_1_7_0/1 -> power15/1(re)
  delay1_1_7_1/1 -> power15/2(im)
  power15/1(re_out) -> ri_to_c1_1_7/1
  power15/2(im_out) -> ri_to_c1_1_7/2
  Constant/1 -> din1_x_din0*/1

== system ami_fx_sbl_wide/ct_tvg1 ==
  enable : Inport
  sync_in : Inport  Port=2
  din : Inport  Port=3
  Concat{1..4} (4 alike) : xbsIndex_r4/Concat  num_inputs=2  dbl_ovrd=off  block_type=concat
  Concat5 : xbsIndex_r4/Concat  num_inputs=4  dbl_ovrd=off  block_type=concat
  Convert{,1..7} (8 alike) : xbsIndex_r4/Convert  gui_display_data_type=Fixed-point  arith_type=Unsigned  n_bits=channel_bits*2  bin_pt=0  float_type=Single  exp_bits=8  fraction_bits=24  quantization=Truncate  overflow=Wrap  en=off  latency=0  dbl_ovrd=off  pipeline=off  block_type=convert
      settings: block_version=11.4
  Counter1 : xbsIndex_r4/Counter  cnt_type=Free Running  cnt_to=10  operation=Up  start_count=2  cnt_by_val=8  arith_type=Unsigned  n_bits=num_channels_bits  bin_pt=0  load_pin=off  rst=on  en=off  explicit_period=on  period=1  dbl_ovrd=off  use_behavioral_HDL=off  implementation=Fabric  block_type=counter
      settings: block_version=11.4
  Counter2 : xbsIndex_r4/Counter  cnt_type=Free Running  cnt_to=10  operation=Up  start_count=0  cnt_by_val=8  arith_type=Unsigned  n_bits=num_channels_bits  bin_pt=0  load_pin=off  rst=on  en=off  explicit_period=on  period=1  dbl_ovrd=off  use_behavioral_HDL=off  implementation=Fabric  block_type=counter
      settings: block_version=11.4
  Counter3 : xbsIndex_r4/Counter  cnt_type=Free Running  cnt_to=10  operation=Up  start_count=3  cnt_by_val=8  arith_type=Unsigned  n_bits=num_channels_bits  bin_pt=0  load_pin=off  rst=on  en=off  explicit_period=on  period=1  dbl_ovrd=off  use_behavioral_HDL=off  implementation=Fabric  block_type=counter
      settings: block_version=11.4
  Counter4 : xbsIndex_r4/Counter  cnt_type=Free Running  cnt_to=10  operation=Up  start_count=1  cnt_by_val=8  arith_type=Unsigned  n_bits=num_channels_bits  bin_pt=0  load_pin=off  rst=on  en=off  explicit_period=on  period=1  dbl_ovrd=off  use_behavioral_HDL=off  implementation=Fabric  block_type=counter
      settings: block_version=11.4
  Counter5 : xbsIndex_r4/Counter  cnt_type=Free Running  cnt_to=10  operation=Up  start_count=6  cnt_by_val=8  arith_type=Unsigned  n_bits=num_channels_bits  bin_pt=0  load_pin=off  rst=on  en=off  explicit_period=on  period=1  dbl_ovrd=off  use_behavioral_HDL=off  implementation=Fabric  block_type=counter
      settings: block_version=11.4
  Counter6 : xbsIndex_r4/Counter  cnt_type=Free Running  cnt_to=10  operation=Up  start_count=4  cnt_by_val=8  arith_type=Unsigned  n_bits=num_channels_bits  bin_pt=0  load_pin=off  rst=on  en=off  explicit_period=on  period=1  dbl_ovrd=off  use_behavioral_HDL=off  implementation=Fabric  block_type=counter
      settings: block_version=11.4
  Counter7 : xbsIndex_r4/Counter  cnt_type=Free Running  cnt_to=10  operation=Up  start_count=7  cnt_by_val=8  arith_type=Unsigned  n_bits=num_channels_bits  bin_pt=0  load_pin=off  rst=on  en=off  explicit_period=on  period=1  dbl_ovrd=off  use_behavioral_HDL=off  implementation=Fabric  block_type=counter
      settings: block_version=11.4
  Counter8 : xbsIndex_r4/Counter  cnt_type=Free Running  cnt_to=10  operation=Up  start_count=5  cnt_by_val=8  arith_type=Unsigned  n_bits=num_channels_bits  bin_pt=0  load_pin=off  rst=on  en=off  explicit_period=on  period=1  dbl_ovrd=off  use_behavioral_HDL=off  implementation=Fabric  block_type=counter
      settings: block_version=11.4
  Delay : xbsIndex_r4/Delay  rst=off  infoeditControl=Selection of Reset will increase slice count due to use of real FFs and instead of SRLs  en=off  latency=1  dbl_ovrd=off  reg_retiming=off  block_type=delay
      settings: block_version=11.4
  Mux1 : xbsIndex_r4/Mux  inputs=2  en=off  latency=1  precision=Full  arith_type=Unsigned  n_bits=16  bin_pt=14  quantization=Truncate  overflow=Wrap  dbl_ovrd=off  block_type=mux
      settings: block_version=11.4
  sync_out : Outport
  dout : Outport  Port=2
  wires:
  Counter2/1 -> Convert/1
  Counter4/1 -> Convert1/1
  sync_in/1 -> Counter2/1, Delay/1, Counter7/1, Counter5/1, Counter8/1, Counter6/1, Counter3/1, Counter1/1, Counter4/1
  Mux1/1 -> dout/1
  enable/1 -> Mux1/1
  din/1 -> Mux1/2
  Convert/1 -> Concat1/1
  Convert1/1 -> Concat1/2
  Delay/1 -> sync_out/1
  Convert2/1 -> Concat2/1
  Counter1/1 -> Convert2/1
  Counter3/1 -> Convert3/1
  Counter6/1 -> Convert4/1
  Counter8/1 -> Convert5/1
  Counter5/1 -> Convert6/1
  Counter7/1 -> Convert7/1
  Concat2/1 -> Concat5/2
  Concat3/1 -> Concat5/3
  Concat1/1 -> Concat5/1
  Concat4/1 -> Concat5/4
  Concat5/1 -> Mux1/3
  Convert3/1 -> Concat2/2
  Convert4/1 -> Concat3/1
  Convert5/1 -> Concat3/2
  Convert6/1 -> Concat4/1
  Convert7/1 -> Concat4/2

== system ami_fx_sbl_wide/ct_tvg2 ==
  enable : Inport
  sync_in : Inport  Port=2
  din : Inport  Port=3
  Concat{1..4} (4 alike) : xbsIndex_r4/Concat  num_inputs=2  dbl_ovrd=off  block_type=concat
  Concat5 : xbsIndex_r4/Concat  num_inputs=4  dbl_ovrd=off  block_type=concat
  Convert{,1..7} (8 alike) : xbsIndex_r4/Convert  gui_display_data_type=Fixed-point  arith_type=Unsigned  n_bits=channel_bits*2  bin_pt=0  float_type=Single  exp_bits=8  fraction_bits=24  quantization=Truncate  overflow=Wrap  en=off  latency=0  dbl_ovrd=off  pipeline=off  block_type=convert
      settings: block_version=11.4
  Counter1 : xbsIndex_r4/Counter  cnt_type=Free Running  cnt_to=10  operation=Up  start_count=2  cnt_by_val=8  arith_type=Unsigned  n_bits=num_channels_bits  bin_pt=0  load_pin=off  rst=on  en=off  explicit_period=on  period=1  dbl_ovrd=off  use_behavioral_HDL=off  implementation=Fabric  block_type=counter
      settings: block_version=11.4
  Counter2 : xbsIndex_r4/Counter  cnt_type=Free Running  cnt_to=10  operation=Up  start_count=0  cnt_by_val=8  arith_type=Unsigned  n_bits=num_channels_bits  bin_pt=0  load_pin=off  rst=on  en=off  explicit_period=on  period=1  dbl_ovrd=off  use_behavioral_HDL=off  implementation=Fabric  block_type=counter
      settings: block_version=11.4
  Counter3 : xbsIndex_r4/Counter  cnt_type=Free Running  cnt_to=10  operation=Up  start_count=3  cnt_by_val=8  arith_type=Unsigned  n_bits=num_channels_bits  bin_pt=0  load_pin=off  rst=on  en=off  explicit_period=on  period=1  dbl_ovrd=off  use_behavioral_HDL=off  implementation=Fabric  block_type=counter
      settings: block_version=11.4
  Counter4 : xbsIndex_r4/Counter  cnt_type=Free Running  cnt_to=10  operation=Up  start_count=1  cnt_by_val=8  arith_type=Unsigned  n_bits=num_channels_bits  bin_pt=0  load_pin=off  rst=on  en=off  explicit_period=on  period=1  dbl_ovrd=off  use_behavioral_HDL=off  implementation=Fabric  block_type=counter
      settings: block_version=11.4
  Counter5 : xbsIndex_r4/Counter  cnt_type=Free Running  cnt_to=10  operation=Up  start_count=6  cnt_by_val=8  arith_type=Unsigned  n_bits=num_channels_bits  bin_pt=0  load_pin=off  rst=on  en=off  explicit_period=on  period=1  dbl_ovrd=off  use_behavioral_HDL=off  implementation=Fabric  block_type=counter
      settings: block_version=11.4
  Counter6 : xbsIndex_r4/Counter  cnt_type=Free Running  cnt_to=10  operation=Up  start_count=4  cnt_by_val=8  arith_type=Unsigned  n_bits=num_channels_bits  bin_pt=0  load_pin=off  rst=on  en=off  explicit_period=on  period=1  dbl_ovrd=off  use_behavioral_HDL=off  implementation=Fabric  block_type=counter
      settings: block_version=11.4
  Counter7 : xbsIndex_r4/Counter  cnt_type=Free Running  cnt_to=10  operation=Up  start_count=7  cnt_by_val=8  arith_type=Unsigned  n_bits=num_channels_bits  bin_pt=0  load_pin=off  rst=on  en=off  explicit_period=on  period=1  dbl_ovrd=off  use_behavioral_HDL=off  implementation=Fabric  block_type=counter
      settings: block_version=11.4
  Counter8 : xbsIndex_r4/Counter  cnt_type=Free Running  cnt_to=10  operation=Up  start_count=5  cnt_by_val=8  arith_type=Unsigned  n_bits=num_channels_bits  bin_pt=0  load_pin=off  rst=on  en=off  explicit_period=on  period=1  dbl_ovrd=off  use_behavioral_HDL=off  implementation=Fabric  block_type=counter
      settings: block_version=11.4
  Delay : xbsIndex_r4/Delay  rst=off  infoeditControl=Selection of Reset will increase slice count due to use of real FFs and instead of SRLs  en=off  latency=1  dbl_ovrd=off  reg_retiming=off  block_type=delay
      settings: block_version=11.4
  Mux1 : xbsIndex_r4/Mux  inputs=2  en=off  latency=1  precision=Full  arith_type=Unsigned  n_bits=16  bin_pt=14  quantization=Truncate  overflow=Wrap  dbl_ovrd=off  block_type=mux
      settings: block_version=11.4
  sync_out : Outport
  dout : Outport  Port=2
  wires:
  Convert7/1 -> Concat4/2
  Convert6/1 -> Concat4/1
  Convert5/1 -> Concat3/2
  Convert4/1 -> Concat3/1
  Convert3/1 -> Concat2/2
  Concat5/1 -> Mux1/3
  Concat4/1 -> Concat5/4
  Concat1/1 -> Concat5/1
  Concat3/1 -> Concat5/3
  Concat2/1 -> Concat5/2
  Counter7/1 -> Convert7/1
  Counter5/1 -> Convert6/1
  Counter8/1 -> Convert5/1
  Counter6/1 -> Convert4/1
  Counter3/1 -> Convert3/1
  Counter1/1 -> Convert2/1
  Convert2/1 -> Concat2/1
  Delay/1 -> sync_out/1
  Convert1/1 -> Concat1/2
  Convert/1 -> Concat1/1
  din/1 -> Mux1/2
  enable/1 -> Mux1/1
  Mux1/1 -> dout/1
  sync_in/1 -> Counter4/1, Counter1/1, Counter3/1, Counter6/1, Counter8/1, Counter5/1, Counter7/1, Delay/1, Counter2/1
  Counter4/1 -> Convert1/1
  Counter2/1 -> Convert/1
